simulink model "tank"  (R2014a)
settings: Solver=ode1  StartTime=0.0  StopTime=inf  FixedStep=delta_t  RelTol=1e-3
PreLoadFcn:
  | model_prediction_init
values from neighbouring files (symbols this model uses):
  C_plant = [1 2]    [model_prediction_init.m]
  delta_t = 0.001    [model_prediction_init.m]
  tank_area = [4 5]    [model_prediction_init.m]
settings Model: CovSFcnEnable=on  BufferReuse=off  Creator=Z133214  LastModifiedBy=kohei-y
settings DataIOCC: SignalLoggingSaveFormat=ModelDataLogs
settings OptimizationCC: BlockReduction=off  BooleanDataType=off  ConditionallyExecuteInputs=off  OptimizeBlockIOStorage=off  BufferReuse=off  GlobalBufferReuse=off  ExpressionFolding=off  ExpressionDepthLimit=2147483647  LocalBlockOutputs=off  OptimizeModelRefInitCode=on  LifeSpan=Inf  SimCompilerOptimization=off
settings DebuggingCC: UnderspecifiedInitializationDetection=Classic  FcnCallInpInsideContextMsg=UseLocalSettings  FrameProcessingCompatibilityMsg=error  StateNameClashWarn=warning
settings RTWCC: SystemTargetFile=ert.tlc  GenCodeOnly=on  TemplateMakefile=ert_default_tmf  Description=Real-Time Workshop Embedded Coder  RTWCompilerOptimization=off
settings CodeAppCC: IgnoreCustomStorageClasses=off  CustomSymbolStrType=$N$R$M  InternalIdentifier=Classic
settings ERTTargetCC: ParMdlRefBuildCompliant=on  CompOptLevelCompliant=on  ConcurrentExecutionCompliant=on  ERTFirstTimeCompliant=on  ModelStepFunctionPrototypeControlCompliant=on  CPPClassGenCompliant=on  InlinedParameterPlacement=Hierarchical  ERTCustomFileTemplate=example_file_process.tlc

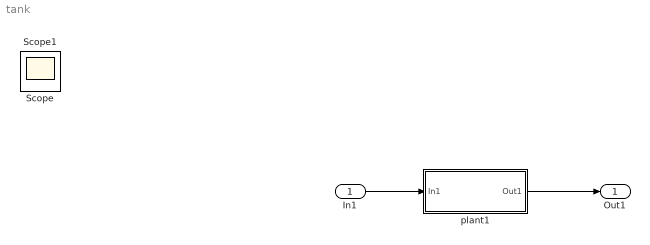
== system tank ==
  In1 : Inport
  plant1 : Subsystem
  Out1 : Outport
  Scope : Scope  NumInputPorts=2
      settings: TimeRange=5  YMin=0~0  YMax=175~4  MaxDataPoints=7500
  Scope1 : Scope
      settings: MaxDataPoints=7500
  wires:
  In1/1 -> plant1/1(In1)
  plant1/1(Out1) -> Out1/1

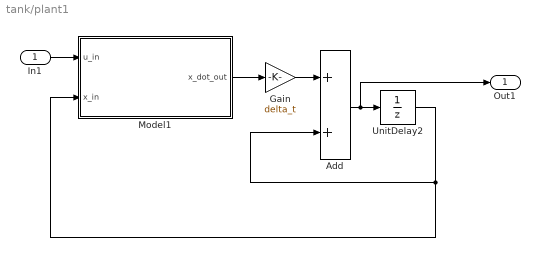
== system tank/plant1 ==
  In1 : Inport
  Add : Sum
  Gain : Gain  Gain=delta_t
  Model1 : Subsystem
  UnitDelay2 : UnitDelay  InitialCondition=[0.01;0.01]  SampleTime=-1
  Out1 : Outport
  wires:
  UnitDelay2/1 -> Model1/2(x_in), Add/2
  In1/1 -> Model1/1(u_in)
  Add/1 -> Out1/1, UnitDelay2/1
  Gain/1 -> Add/1
  Model1/1(x_dot_out) -> Gain/1

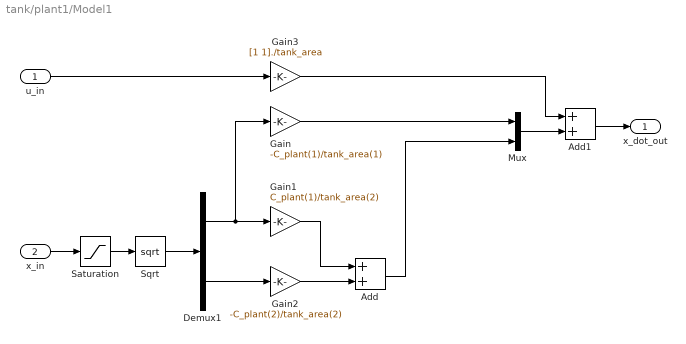
== system tank/plant1/Model1 ==
  u_in : Inport  PortDimensions=realu_dim
  x_in : Inport  Port=2  PortDimensions=x_dim
  Add : Sum
  Add1 : Sum
  Demux1 : Demux  Outputs=2
  Gain : Gain  Gain=-C_plant(1)/tank_area(1)
  Gain1 : Gain  Gain=C_plant(1)/tank_area(2)
  Gain2 : Gain  Gain=-C_plant(2)/tank_area(2)
  Gain3 : Gain  Gain=[1 1]./tank_area
  Mux : Mux  Inputs=2
  Saturation : Saturate  UpperLimit=inf  LowerLimit=0
  Sqrt : Sqrt  SaturateOnIntegerOverflow=on
  x_dot_out : Outport
  wires:
  Add1/1 -> x_dot_out/1
  x_in/1 -> Saturation/1
  Saturation/1 -> Sqrt/1
  u_in/1 -> Gain3/1
  Mux/1 -> Add1/2
  Gain3/1 -> Add1/1
  Add/1 -> Mux/2
  Gain/1 -> Mux/1
  Gain2/1 -> Add/2
  Gain1/1 -> Add/1
  Demux1/2 -> Gain2/1
  Demux1/1 -> Gain1/1, Gain/1
  Sqrt/1 -> Demux1/1
